simulink model "Quadcopter"  (R2018a)
settings: Solver=VariableStepAuto  StartTime=0.0  StopTime=100.0  RelTol=1e-3
libraries: vrlib x2, simulink x1, realtime_pacer_lib x1
settings Model: Creator=Jarvis  LastModifiedBy=Jarvis

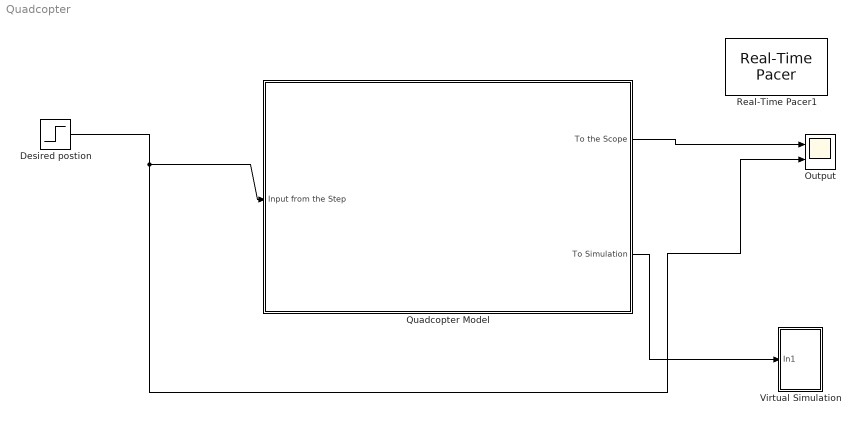
== system Quadcopter ==
  Desired postion : Step  After=2  SampleTime=0
  Output : Scope  NumInputPorts=2
  Quadcopter Model : Subsystem
  Real-Time Pacer1 : realtime_pacer_lib/Real-Time Pacer  simTimePerRealTime=1
  Virtual Simulation : Subsystem
  wires:
  Desired postion/1 -> Output/2, Quadcopter Model/1(Input from the Step)
  Quadcopter Model/1(To the Scope) -> Output/1
  Quadcopter Model/2(To Simulation) -> Virtual Simulation/1(In1)

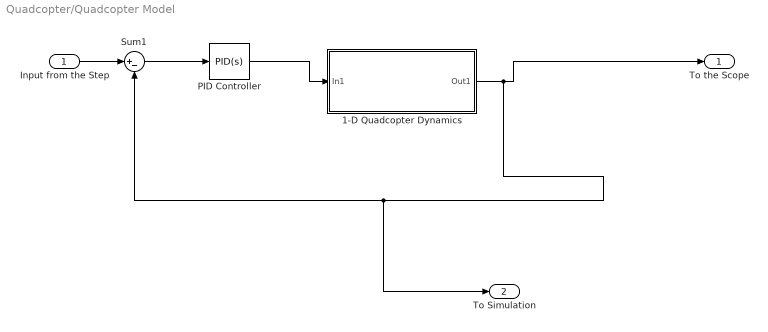
== system Quadcopter/Quadcopter Model ==
  Input from the Step : Inport
  1-D Quadcopter Dynamics : Subsystem
  PID Controller : simulink/Continuous/PID Controller  Controller=PID  TimeDomain=Continuous-time  SampleTime=-1  IntegratorMethod=Forward Euler  FilterMethod=Forward Euler  Form=Parallel  UseFilter=on  ControllerParametersSource=internal  P=2.91995946059059  I=0.321025602189606  D=6.20958419018746  N=352.873116541379  InitialConditionSource=internal  InitialConditionForIntegrator=0  InitialConditionForFilter=0  ExternalReset=none  LimitOutput=off  UpperSaturationLimit=inf  LowerSaturationLimit=-inf  LinearizeAsGain=on  AntiWindupMode=none  Kb=1  TrackingMode=off  Kt=1  PParamMin=[]  PParamMax=[]  IParamMin=[]  IParamMax=[]  DParamMin=[]  DParamMax=[]  NParamMin=[]  NParamMax=[]  KbParamMin=[]  KbParamMax=[]  KtParamMin=[]  KtParamMax=[]  POutMin=[]  POutMax=[]  IOutMin=[]  IOutMax=[]  DOutMin=[]  DOutMax=[]  NOutMin=[]  NOutMax=[]  KbOutMin=[]  KbOutMax=[]  KtOutMin=[]  KtOutMax=[]  IntegratorOutMin=[]  IntegratorOutMax=[]  FilterOutMin=[]  FilterOutMax=[]  SumOutMin=[]  SumOutMax=[]  SumI1OutMin=[]  SumI1OutMax=[]  SumI2OutMin=[]  SumI2OutMax=[]  SumI3OutMin=[]  SumI3OutMax=[]  SumDOutMin=[]  SumDOutMax=[]  SaturationOutMin=[]  SaturationOutMax=[]  IntegratorContinuousStateAttributes=''  IntegratorStateMustResolveToSignalObject=off  IntegratorRTWStateStorageClass=Auto  FilterContinuousStateAttributes=''  FilterStateMustResolveToSignalObject=off  FilterRTWStateStorageClass=Auto  DifferentiatorICPrevScaledInput=0  DifferentiatorOutMin=[]  DifferentiatorOutMax=[]  FilterDiffOutCoefMin=[]  FilterDiffOutCoefMax=[]  SumDenOutMin=[]  SumDenOutMax=[]  SumNumOutMin=[]  SumNumOutMax=[]  ReciprocalOutMin=[]  ReciprocalOutMax=[]  DivideOutMin=[]  DivideOutMax=[]  TunerSelectOption=Transfer Function Based (PID Tuner App)
  Sum1 : Sum  Inputs=|+-
  To the Scope : Outport
  To Simulation : Outport  Port=2
  wires:
  Sum1/1 -> PID Controller/1
  PID Controller/1 -> 1-D Quadcopter Dynamics/1(In1)
  Input from the Step/1 -> Sum1/1
  1-D Quadcopter Dynamics/1(Out1) -> To Simulation/1, Sum1/2, To the Scope/1

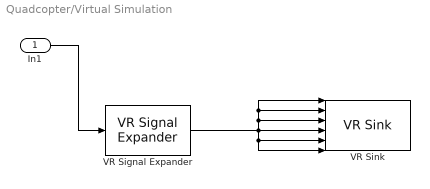
== system Quadcopter/Virtual Simulation ==
  In1 : Inport
  VR Signal Expander : vrlib/VR Signal Expander  outwidth=3  outidx=[2]
      settings: SourceProductName=Simulink 3D Animation  SourceProductBaseCode=VR
  VR Sink : vrlib/VR Sink  InstantiateOnLoad=on  SampleTime=0.01  ViewEnable=on  RemoteChange=off  RemoteView=off  FieldsWritten=Fan_1.translation.3.1.1.double#Fan_2.translation.3.1.1.double#Fan_3.translation.3.1.1.double#Fan_4.translation.3.1.1.double#z_arm.translation.3.1.1.double#x_arm.translation.3.1.1.double  WorldFileName=QuadCopter.wrl  AutoView=off  VideoDimensions=[]  AllowVariableSize=off
      settings: SourceProductBaseCode=VR
  wires:
  In1/1 -> VR Signal Expander/1
  VR Signal Expander/1 -> VR Sink/6, VR Sink/5, VR Sink/3, VR Sink/2, VR Sink/1, VR Sink/4

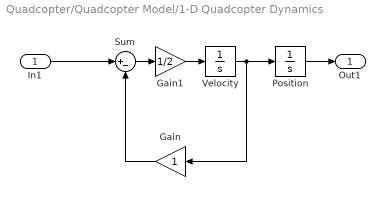
== system Quadcopter/Quadcopter Model/1-D Quadcopter Dynamics ==
  In1 : Inport
  Gain : Gain
  Gain1 : Gain  Gain=1/2
  Position : Integrator
  Sum : Sum  Inputs=|+-
  Velocity : Integrator
  Out1 : Outport
  wires:
  Gain/1 -> Sum/2
  Velocity/1 -> Position/1, Gain/1
  In1/1 -> Sum/1
  Sum/1 -> Gain1/1
  Position/1 -> Out1/1
  Gain1/1 -> Velocity/1
